simulink model "Matlab_2023_Betta_Photovoltaic_Environmental_Effects"  (R2023b)
settings: Solver=VariableStepAuto  StartTime=0.0  StopTime=60*10*6  RelTol=1e-3  EnableMultiTasking=on
PreLoadFcn:
  | initial_temperature = 20;
  | v_ac_nom = 110;
  | 
  | % Properties for each of the series-connected
  | % set of panels
  | area = 9;
  | thickness = 0.003;
  | cp = 840;
  | 
  | % Optimum operating point obtained from
  | % running SolarCellPowerCurveExample
  | if ~exist('voltageTable','var')
  |     voltageTable = [
  |       308.3333  275.0000
  |       329.1667  295.8333
  |       341.6667  312.5000];
  |     irradianceVec =[200 500 1000];
  |     temperatureVec =[20 40];
  | end
  | 
  | load PhotovoltaicGeneratorPVMaxPowerMap
libraries: fl_lib x12, nesl_utility x7, fl_ps_legacy_lib x6, ee_lib x2, SignalEditorBlockLib x1
CloseFcn:
  | try,close(h1_PhotovoltaicGenerator),end
  | clear h1_PhotovoltaicGenerator
  | try,close(h2_PhotovoltaicGenerator),end
  | clear h2_PhotovoltaicGenerator
  | 
  | 
  | clear simlog_PhotovoltaicGenerator
  | clear logsout_PhotovoltaicGenerator
  | clear PVMaxPowerMap area cp initial_temperature irradianceVec temperatureVec thickness v_ac_nom voltageTable
Description:
  | Photovoltaic Generator
settings Model: Creator=The MathWorks, Inc.
settings SolverCC: AlgebraicLoopSolver=TrustRegion
settings DataIOCC: MaxDataPoints=10000  SaveFormat=Array  SaveOutput=off  SignalLogging=off  DSMLogging=off  SaveTime=off  ReturnWorkspaceOutputs=off  SignalLoggingName=logsout_PhotovoltaicGenerator  OutputTimes=[0:0.005:60]
settings OptimizationCC: ReuseModelBlockBuffer=off  ExpressionDepthLimit=2147483647  LifeSpan=inf
settings DebuggingCC: UnderspecifiedInitializationDetection=Classic  MergeDetectMultiDrivingBlocksExec=none  FcnCallInpInsideContextMsg=warning  UnconnectedInputMsg=warning  UnconnectedOutputMsg=warning  UnconnectedLineMsg=warning  StateNameClashWarn=warning  SFUnexpectedBacktrackingDiag=warning  SFNoUnconditionalDefaultTransitionDiag=warning  SFExecutionAtInitializationDiag=none  ArithmeticOperatorsInVariantConditions=warning
settings HardwareCC: ProdBitPerPointer=32  ProdBitPerSizeT=32  ProdBitPerPtrDiffT=32  ProdLargestAtomicFloat=None  ProdIntDivRoundTo=Undefined  ProdEndianess=Unspecified  ProdWordSize=32  ProdHWDeviceType=32-bit Generic
settings ModelReferenceCC: EnableRefExpFcnMdlSchedulingChecks=on  PropagateSignalLabelsOutOfModel=off
settings SFSimCC: SimUseLocalCustomCode=off  CustomCodeUndefinedFunction=UseInterfaceOnly
settings RTWCC: RTWUseLocalCustomCode=off  DLArmComputeVersion=19.05
settings CodeAppCC: StateflowObjectComments=on
settings GRTTargetCC: TargetLangStandard=C89/C90 (ANSI)  CombineOutputUpdateFcns=off  GRTInterface=on
settings ConfigComp: CovMetricSettings=dw  CovSaveCumulativeToWorkspaceVar=on  CovSaveSingleToWorkspaceVar=on  CovExternalEMLEnable=off  CovSFcnEnable=off
settings SimscapeCC: SimscapeLogType=all  SimscapeLogSimulationStatistics=on  SimscapeLogName=simlog_PhotovoltaicGenerator  SimscapeLogDataHistory=10000

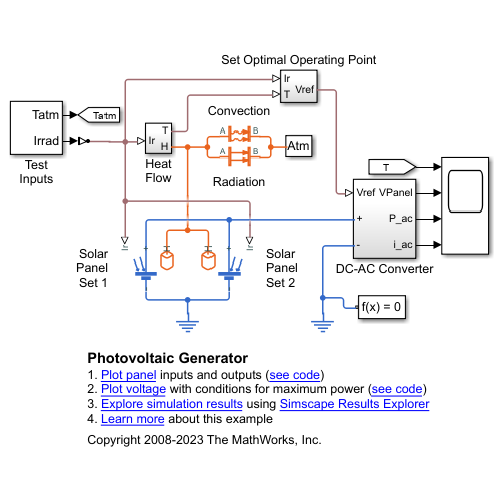
[thumbnail: Simulink's stored preview of the top-level diagram]
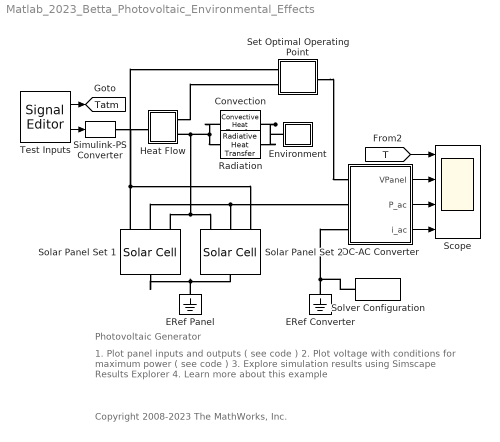
== system Matlab_2023_Betta_Photovoltaic_Environmental_Effects ==
  note: Photovoltaic Generator
  note: 1. Plot panel inputs and outputs ( see code )
      | 2. Plot voltage with conditions for maximum power ( see code )
      | 3. Explore simulation results using Simscape Results Explorer
      | 4. Learn more about this example
  note: Copyright 2008-2023 The MathWorks, Inc.
  Convection : fl_lib/Thermal/Thermal Elements/Convective Heat Transfer  thermal_type=foundation.enum.constant_variable.constant  area=2*area m^2  heat_tr_coeff=20 W/(m^2 * K)  min_heat_tr_coeff=1e-3 W/(K*m^2)  T_specify=off  T_priority=High  T=0 K  T_nominal_specify=off  T_nominal_unit=K  T_nominal_value=1  Q_specify=off  Q_priority=High  Q=0 J/s  Q_nominal_specify=off  Q_nominal_unit=J/s  Q_nominal_value=1
  DC-AC Converter : Subsystem
  ERef Converter : fl_lib/Electrical/Electrical Elements/Electrical Reference
  ERef Panel : fl_lib/Electrical/Electrical Elements/Electrical Reference
  Environment : Subsystem
      mask Display: disp('Atm')
  Heat Flow : Subsystem
  Radiation : fl_lib/Thermal/Thermal Elements/Radiative Heat Transfer  area=2*area m^2  rad_tr_coeff=2e-8 W/(m^2*K^4)  T_specify=off  T_priority=High  T=0 K  T_nominal_specify=off  T_nominal_unit=K  T_nominal_value=1  Q_specify=off  Q_priority=High  Q=0 J/s  Q_nominal_specify=off  Q_nominal_unit=J/s  Q_nominal_value=1
      settings: InternalSimscapePortConfiguration="{\"Bottom\":[],\"Left\":[{\"id\":\"A\",\"label\":\"A\",\"type\":\"foundation.thermal.thermal\"}],\"Right\":[{\"id\":\"B\",\"label\":\"B\",\"type\":\"foundation.thermal.thermal\"}],\"Top\":[]}"
  Scope : Scope  NumInputPorts=4
  Set Optimal Operating Point : Subsystem
  Simulink-PS Converter : nesl_utility/Simulink-PS Converter  PhysicalDomain=network_engine_domain  SubClassName=ps_input  LeftPortType=input  RightPortType=output  PseudoPeriodic=off  Frequencies=[]  NoiseDistribution=none  NoiseParameters=[]  Unit=1  AffineConversion=off  FilteringAndDerivatives=filter  SimscapeFilterOrder=1  InputFilterTimeConstant=1  UdotUserProvided=1
  Solar Panel Set 1 : ee_lib/Sources/Solar Cell  prm=3  Isc=3.8 A  Voc=0.586 V  Is=3.15e-07 A  Is2=0 A  Iph=3.80 A  Ir0=1000 W/m^2  ec=1.4  N2=2  Rs=0.0042 Ohm  Rp=10.1 Ohm  N_series=700  N_parallel=1  TIPH1=0.000805 1/K  EG=1.14 eV  TXIS1=3.38  TXIS2=3  TRS1=0  TRP1=0  Tmeas=25 degC  TFIXED=25 degC  thermal_mass=area*thickness*cp J/K  initial_temperature=initial_temperature degC
      settings: InternalSimscapePortConfiguration="{\"Bottom\":[],\"Left\":[{\"id\":\"Ir\",\"label\":\"Ir\",\"type\":\"input\"},{\"id\":\"p\",\"label\":\"+\",\"type\":\"foundation.electrical.electrical\"},{\"id\":\"H\",\"label\":\"H\",\"type\":\"foundation.thermal.thermal\"}],\"Right\":[{\"id\":\"n\",\"label\":\"-\",\"type\":\"foundation.electrical.electrical\"}],\"Top\":[]}"
  Solar Panel Set 2 : ee_lib/Sources/Solar Cell  prm=3  Isc=3.8 A  Voc=0.586 V  Is=3.15e-07 A  Is2=0 A  Iph=3.80 A  Ir0=1000 W/m^2  ec=1.4  N2=2  Rs=0.0042 Ohm  Rp=10.1 Ohm  N_series=700  N_parallel=1  TIPH1=0.000805 1/K  EG=1.14 eV  TXIS1=3.38  TXIS2=3  TRS1=0  TRP1=0  Tmeas=25 degC  TFIXED=25 degC  thermal_mass=area*thickness*cp J/K  initial_temperature=initial_temperature degC
      settings: InternalSimscapePortConfiguration="{\"Bottom\":[],\"Left\":[{\"id\":\"Ir\",\"label\":\"Ir\",\"type\":\"input\"},{\"id\":\"p\",\"label\":\"+\",\"type\":\"foundation.electrical.electrical\"},{\"id\":\"H\",\"label\":\"H\",\"type\":\"foundation.thermal.thermal\"}],\"Right\":[{\"id\":\"n\",\"label\":\"-\",\"type\":\"foundation.electrical.electrical\"}],\"Top\":[]}"
  Solver Configuration : nesl_utility/Solver Configuration  PhysicalDomain=network_engine_domain  SubClassName=solver  LeftPortType=input  RightPortType=generic  Tones=[]  Harmonics=[]  SimulateNoise=off  Profile=off  UseLocalSampling=off  EnableSwitchedLinearOptims=on  FrequencyDomain=off  UseCCode=off  RelTol=0.001  AbsTol=1e-06  MinStep=1e-09  ToWorkspace=off  RevertToSquareIcSolve=off  NumHomotopyIterations=100  PhasorMode=off  PhasorModeNumHarmonics=1  ConsistencySolver=NEWTON_FTOL  IndexReductionMethod=DerivativeReplacement  DoDC=on  ResidualTolerance=1e-9  ConsistencyTolSource=GLOBAL  ConsistencyAbsTol=0.001  ConsistencyRelTol=0.001  ConsistencyTolFactor=0.001  UseLocalSolver=off  LocalSolverChoice=NE_TRAPEZOIDAL_ADVANCER  ResolveIndetEquations=on  FunctionEvalNumThread=1  LocalSolverSampleTime=1e-7  DoFixedCost=off  MaxNonlinIter=10  MaxModeIter=2  ComputeImpulses=off  ImpulseIterations=1  LinearAlgebra=auto  LinearAlgebraNumThread=0  EquationFormulation=NE_TIME_EF  DelaysMemoryBudget=1024  AutomaticFiltering=on  FilteringTimeConstant=0.001  PartitionStorageMethod=AS_NEEDED  PartitionMemoryBudget=1024  PartitionMethod=FAST  MultibodyUseLocalSolver=off  MultibodyLocalSolverChoice=ODE1  MultibodyLocalSolverSampleTime=0.001
  Test Inputs : SignalEditorBlockLib/Signal Editor  FileName=PhotovoltaicGeneratorTestInputs.mat  ActiveScenario=Group_1  ActiveSignal=Irrad  IsBus=off  OutputBusObjectStr=Bus: BusObject  SampleTime=0  OutputAfterFinalValue=Extrapolation  Unit=inherit  PreserveSignalName=on  ApplySigPropsToAllScenarios=on  ApplySigPropsToAllSignals=off
  tag scope: Tatm=global
  wires:
  Test Inputs/2 -> Simulink-PS Converter/1
  DC-AC Converter/3(i_ac) -> Scope/4
  DC-AC Converter/2(P_ac) -> Scope/3
  [T] -> Scope/1
  DC-AC Converter/1(VPanel) -> Scope/2
  Test Inputs/1 -> [Tatm]
  connections:
  Solar Panel Set 1/LConn2 -- DC-AC Converter/LConn2 -- Solar Panel Set 2/LConn2
  Convection/LConn1 -- Radiation/LConn1 -- Solar Panel Set 2/LConn3 -- Solar Panel Set 1/LConn3 -- Heat Flow/LConn2
  Set Optimal Operating Point/RConn1 -- DC-AC Converter/LConn1
  ERef Panel/LConn1 -- Solar Panel Set 2/RConn1 -- Solar Panel Set 1/RConn1
  ERef Converter/LConn1 -- Solver Configuration/RConn1 -- DC-AC Converter/LConn3
  Heat Flow/LConn1 -- Set Optimal Operating Point/LConn2
  Solar Panel Set 1/LConn1 -- Heat Flow/RConn1 -- Simulink-PS Converter/RConn1 -- Set Optimal Operating Point/LConn1 -- Solar Panel Set 2/LConn1
  Convection/RConn1 -- Radiation/RConn1 -- Environment/LConn1

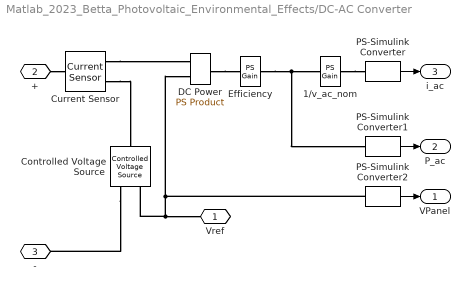
== system Matlab_2023_Betta_Photovoltaic_Environmental_Effects/DC-AC Converter ==
  1/v_ac_nom : fl_ps_legacy_lib/Legacy Physical Signals/Functions/PS Gain  gain=1/v_ac_nom
  Controlled Voltage Source : fl_lib/Electrical/Electrical Sources/Controlled Voltage Source
  Current Sensor : fl_lib/Electrical/Electrical Sensors/Current Sensor
  DC Power : fl_ps_legacy_lib/Legacy Physical Signals/Functions/PS Product
  Efficiency : fl_ps_legacy_lib/Legacy Physical Signals/Functions/PS Gain  gain=0.97
      settings: AttributesFormatString=%<gain>
  PS-Simulink Converter : nesl_utility/PS-Simulink Converter  PhysicalDomain=network_engine_domain  SubClassName=ps_output  LeftPortType=input  RightPortType=output  PseudoPeriodic=off  Frequencies=[]  VectorFormat=1-D array  Unit=A  AffineConversion=off
  PS-Simulink Converter1 : nesl_utility/PS-Simulink Converter  PhysicalDomain=network_engine_domain  SubClassName=ps_output  LeftPortType=input  RightPortType=output  PseudoPeriodic=off  Frequencies=[]  VectorFormat=1-D array  Unit=W  AffineConversion=off
  PS-Simulink Converter2 : nesl_utility/PS-Simulink Converter  PhysicalDomain=network_engine_domain  SubClassName=ps_output  LeftPortType=input  RightPortType=output  PseudoPeriodic=off  Frequencies=[]  VectorFormat=1-D array  Unit=V  AffineConversion=off
  Vref : PMIOPort  Side=Left
  + : PMIOPort  Port=2  Side=Left
  - : PMIOPort  Port=3  Side=Left
  VPanel : Outport  VectorParamsAs1DForOutWhenUnconnected=off
  P_ac : Outport  Port=2  VectorParamsAs1DForOutWhenUnconnected=off
  i_ac : Outport  Port=3  VectorParamsAs1DForOutWhenUnconnected=off
  wires:
  PS-Simulink Converter/1 -> i_ac/1
  PS-Simulink Converter1/1 -> P_ac/1
  PS-Simulink Converter2/1 -> VPanel/1
  connections:
  Controlled Voltage Source/RConn2 -- -/RConn1
  Vref/RConn1 -- Controlled Voltage Source/RConn1 -- PS-Simulink Converter2/LConn1 -- DC Power/LConn2
  +/RConn1 -- Current Sensor/LConn1
  Current Sensor/RConn2 -- Controlled Voltage Source/LConn1
  Current Sensor/RConn1 -- DC Power/LConn1
  DC Power/RConn1 -- Efficiency/LConn1
  Efficiency/RConn1 -- 1/v_ac_nom/LConn1 -- PS-Simulink Converter1/LConn1
  1/v_ac_nom/RConn1 -- PS-Simulink Converter/LConn1

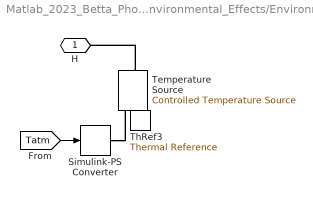
== system Matlab_2023_Betta_Photovoltaic_Environmental_Effects/Environment ==
  Simulink-PS Converter : nesl_utility/Simulink-PS Converter  PhysicalDomain=network_engine_domain  SubClassName=ps_input  LeftPortType=input  RightPortType=output  PseudoPeriodic=off  Frequencies=[]  NoiseDistribution=none  NoiseParameters=[]  Unit=1  AffineConversion=off  FilteringAndDerivatives=zero  SimscapeFilterOrder=1  InputFilterTimeConstant=0.001  UdotUserProvided=1
  Temperature Source : fl_lib/Thermal/Thermal Sources/Controlled Temperature Source
  ThRef3 : fl_lib/Thermal/Thermal Elements/Thermal Reference
  H : PMIOPort  Side=Left
  wires:
  [Tatm] -> Simulink-PS Converter/1
  connections:
  ThRef3/LConn1 -- Temperature Source/RConn2
  Temperature Source/LConn1 -- H/RConn1
  Simulink-PS Converter/RConn1 -- Temperature Source/RConn1

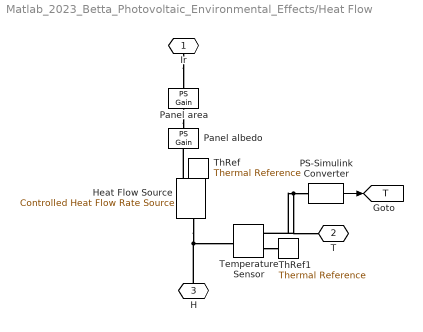
== system Matlab_2023_Betta_Photovoltaic_Environmental_Effects/Heat Flow ==
  Heat Flow Source : fl_lib/Thermal/Thermal Sources/Controlled Heat Flow Rate Source
  PS-Simulink Converter : nesl_utility/PS-Simulink Converter  PhysicalDomain=network_engine_domain  SubClassName=ps_output  LeftPortType=input  RightPortType=output  PseudoPeriodic=off  Frequencies=[]  VectorFormat=1-D array  Unit=degC  AffineConversion=on
  Panel albedo : fl_ps_legacy_lib/Legacy Physical Signals/Functions/PS Gain  gain=0.3
  Panel area : fl_ps_legacy_lib/Legacy Physical Signals/Functions/PS Gain  gain=2*area
  Temperature Sensor : fl_lib/Thermal/Thermal Sensors/Temperature Sensor  temperature_measure=foundation.enum.MeasurementReference.difference
  ThRef : fl_lib/Thermal/Thermal Elements/Thermal Reference
  ThRef1 : fl_lib/Thermal/Thermal Elements/Thermal Reference
  Ir : PMIOPort  Side=Right
  T : PMIOPort  Port=2  Side=Left
  H : PMIOPort  Port=3  Side=Left
  tag scope: T=global
  wires:
  PS-Simulink Converter/1 -> [T]
  connections:
  H/RConn1 -- Temperature Sensor/LConn1 -- Heat Flow Source/LConn1
  PS-Simulink Converter/LConn1 -- Temperature Sensor/RConn2 -- T/RConn1
  Heat Flow Source/RConn1 -- Panel albedo/RConn1
  ThRef/LConn1 -- Heat Flow Source/RConn2
  Ir/RConn1 -- Panel area/LConn1
  Panel area/RConn1 -- Panel albedo/LConn1
  Temperature Sensor/RConn1 -- ThRef1/LConn1

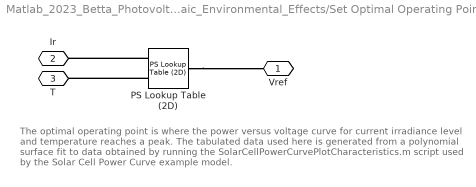
== system Matlab_2023_Betta_Photovoltaic_Environmental_Effects/Set Optimal Operating Point ==
  note: The optimal operating point is where the power versus voltage curve
      | for current irradiance level and temperature reaches a peak. The tabulated
      | data used here is generated from a polynomial surface fit to data obtained
      | by running the SolarCellPowerCurvePlotCharacteristics.m script
      | used by the Solar Cell Power Curve example model.
  PS Lookup Table (2D) : fl_ps_legacy_lib/Legacy Physical Signals/Lookup Tables/PS Lookup Table (2D)  x1=PVMaxPowerMap.iRad_Vect  x2=PVMaxPowerMap.temp_Vect  f=PVMaxPowerMap.VRef_Table'  interp_method=2  extrap_method=1
      settings: InternalSimscapePortConfiguration="{\"Bottom\":[],\"Left\":[{\"id\":\"I1\",\"label\":\"x1\",\"type\":\"input\"},{\"id\":\"I2\",\"label\":\"x2\",\"type\":\"input\"}],\"Right\":[{\"id\":\"O\",\"label\":\"f\",\"type\":\"output\"}],\"Top\":[]}"
  Vref : PMIOPort  Side=Right
  Ir : PMIOPort  Port=2  Side=Left
  T : PMIOPort  Port=3  Side=Left
  connections:
  PS Lookup Table (2D)/RConn1 -- Vref/RConn1
  PS Lookup Table (2D)/LConn1 -- Ir/RConn1
  PS Lookup Table (2D)/LConn2 -- T/RConn1
